simulink model "DC_Motor_w_Load"  (R2019b)
settings: Solver=VariableStepAuto  StartTime=0.0  StopTime=300  RelTol=1e-3
InitFcn:
  | va = 12;   % [V]
  | Ra=7.17;  % [Ohm]
  | k=0.01;      % [N/m]
  | B1=7.05e-5;  % [Nmsec]
  | B2 = 3e-5;       % [Nmsec]
  | J1 = 4.14e-5;    % [kg*m^2]
  | J2 = 2.12e-3;   % [kg*m]
  | ke = 0.29;        % [V*sec]
  | Kt = 4.6e-4;     % [Nm/A]
  | La = 9.53e-4;   % [H]
settings Model: Creator=sulaymon.eshkabilov  LastModifiedBy=sulaymon.eshkabilov

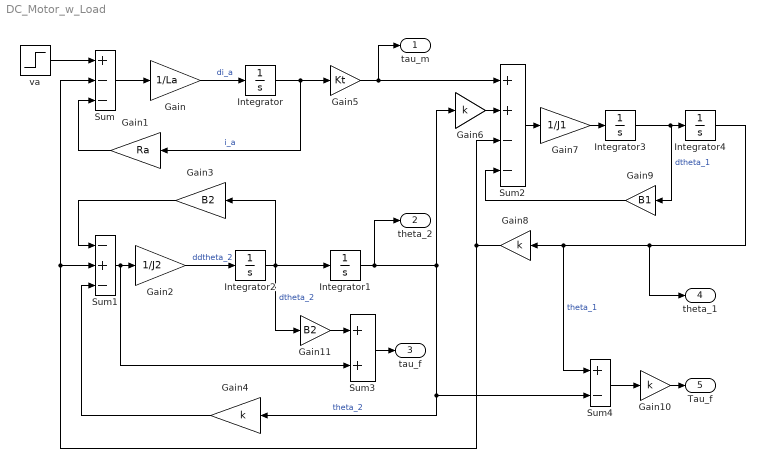
== system DC_Motor_w_Load ==
  Gain : Gain  Gain=1/La
  Gain1 : Gain  Gain=Ra
  Gain{4,6,8,10} (4 alike) : Gain  Gain=k
  Gain11 : Gain  Gain=B2
  Gain2 : Gain  Gain=1/J2
  Gain3 : Gain  Gain=B2
  Gain5 : Gain  Gain=Kt
  Gain7 : Gain  Gain=1/J1
  Gain9 : Gain  Gain=B1
  Integrator{,1..4} (5 alike) : Integrator
  Sum : Sum  Inputs=+--
  Sum1 : Sum  Inputs=-+-
  Sum2 : Sum  Inputs=++--
  Sum3 : Sum
  Sum4 : Sum  Inputs=+-
  va : Step  After=va  SampleTime=0
  tau_m : Outport
  theta_2 : Outport  Port=2
  tau_f : Outport  Port=3
  theta_1 : Outport  Port=4
  Tau_f : Outport  Port=5
  wires:
  Sum/1 -> Gain/1
  Gain/1 -> Integrator/1  "di_a"
  Integrator/1 -> Gain5/1, Gain1/1  "i_a"
  va/1 -> Sum/1
  Gain1/1 -> Sum/3
  Gain2/1 -> Integrator2/1  "ddtheta_2"
  Sum1/1 -> Sum3/2, Gain2/1
  Gain3/1 -> Sum1/1
  Integrator1/1 -> theta_2/1, Sum4/2, Gain4/1, Gain6/1  "theta_2"
  Gain4/1 -> Sum1/3
  Gain5/1 -> Sum2/1, tau_m/1
  Gain6/1 -> Sum2/2
  Sum2/1 -> Gain7/1
  Gain7/1 -> Integrator3/1
  Integrator4/1 -> theta_1/1, Sum4/1, Gain8/1  "theta_1"
  Gain9/1 -> Sum2/4
  Gain8/1 -> Sum/2, Sum1/2, Sum2/3
  Gain11/1 -> Sum3/1
  Sum3/1 -> tau_f/1
  Integrator3/1 -> Gain9/1, Integrator4/1  "dtheta_1"
  Integrator2/1 -> Integrator1/1, Gain11/1, Gain3/1  "dtheta_2"
  Sum4/1 -> Gain10/1
  Gain10/1 -> Tau_f/1
